simulink model "B3"  (R2016a)
settings: Solver=VariableStepAuto  StartTime=0.0  StopTime=10000  RelTol=1e-3
libraries: simulink x1
settings Model: Creator=user  LastModifiedBy=user

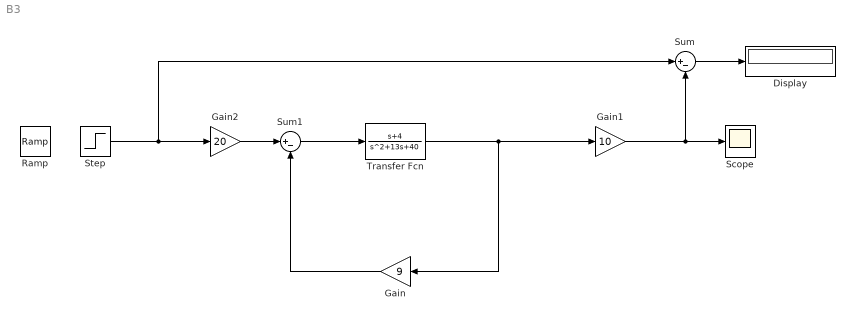
== system B3 ==
  Display : Display
  Gain : Gain  Gain=9
  Gain1 : Gain  Gain=10
  Gain2 : Gain  Gain=20
  Ramp : simulink/Sources/Ramp  slope=1  start=5  X0=0
  Scope : Scope
  Step : Step  Time=0  After=5  SampleTime=0
  Sum : Sum  Inputs=|+-
  Sum1 : Sum  Inputs=|+-
  Transfer Fcn : TransferFcn  Numerator=[1 4]  Denominator="[1 13  40]"
  wires:
  Sum1/1 -> Transfer Fcn/1
  Transfer Fcn/1 -> Gain1/1, Gain/1
  Sum/1 -> Display/1
  Gain1/1 -> Scope/1, Sum/2
  Gain/1 -> Sum1/2
  Gain2/1 -> Sum1/1
  Step/1 -> Sum/1, Gain2/1
